simulink model "UAV"  (R2025b)
settings: Solver=ode3  StartTime=0.0  StopTime=inf  FixedStep=Sim.Ts_fisica  RelTol=1e-3
PostLoadFcn:
  | Init
InitFcn:
  | Init
model workspace (MAT data in the model file):
  Mass = 1
undefined symbols (not defined in the file): DiscIntNeverNeededParam, Drone, DWORK0, DWORK1, DWORK10, DWORK11, DWORK12, DWORK13, DWORK14, DWORK15, DWORK16, DWORK17, DWORK18, DWORK19, DWORK2, DWORK20, DWORK21, DWORK22, DWORK23, DWORK24, DWORK3, DWORK4, DWORK5, DWORK6, DWORK7, DWORK8, DWORK9, F, Light, MIL, Sim
libraries: simulink x35, slpidlib x11, vrlib x4, aerolibwind2 x2, sim3dlib x2, uavsim3dlib x2
(part 7 of 8)

== system UAV/Flight Controller Software/Flight Controller Software MIL/Mix Quad-X ==
  Fz : Inport
  T_Phi : Inport  Port=2
  T_Psi : Inport  Port=3
  T_Theta : Inport  Port=4
  M1 : Sum  Inputs=+---
  M2 : Sum  Inputs=+-++
  M3 : Sum  Inputs=++-+
  M4 : Sum  Inputs=+++-
  Saturation{,1..3} (4 alike) : Saturate  UpperLimit=1  LowerLimit=0
  Sqrt{,1..3} (4 alike) : Sqrt
  Motor 1 : Outport
  Motor 2 : Outport  Port=2
  Motor 3 : Outport  Port=3
  Motor 4 : Outport  Port=4
  wires:
  Fz/1 -> M4/1, M3/1, M2/1, M1/1
  T_Phi/1 -> M4/2, M3/2, M2/2, M1/2
  T_Theta/1 -> M4/3, M3/3, M2/3, M1/3
  T_Psi/1 -> M4/4, M3/4, M2/4, M1/4
  M1/1 -> Saturation/1
  M2/1 -> Saturation1/1
  M3/1 -> Saturation2/1
  M4/1 -> Saturation3/1
  Saturation/1 -> Sqrt/1
  Saturation1/1 -> Sqrt1/1
  Saturation2/1 -> Sqrt2/1
  Saturation3/1 -> Sqrt3/1
  Sqrt/1 -> Motor 1/1
  Sqrt1/1 -> Motor 2/1
  Sqrt2/1 -> Motor 3/1
  Sqrt3/1 -> Motor 4/1

== system UAV/Flight Controller Software/Flight Controller Software MIL/State Estimator ==
  " System_Ready" : Inport
  " " : Inport  Port=2
  Bus Selector : BusSelector  OutputSignals=Wb_m,Acc_m,Mag_m,Xe_m,Ve_m,z_m
  MATLAB Function : MATLAB Function  TreatAsAtomicUnit=on  SystemSampleTime=Sim.Ts_pos
  MATLAB Function2 : MATLAB Function  TreatAsAtomicUnit=on  SystemSampleTime=Sim.Ts_control
  Rate Transition{1..4} (4 alike) : RateTransition  OutPortSampleTime=Sim.Ts_pos
  Selector : Selector  InputPortWidth=6  IndexOptions=Index vector (dialog)  Indices=[3]  OutputSizes=1
  Subsystem : Subsystem
  Transpose : Math  Operator=transpose
  Rates : Outport
  Angles : Outport  Port=2
  Pos : Outport  Port=3
  Vel : Outport  Port=4
  DCMbe : Outport  Port=5
  wires:
  Bus Selector/4 -> MATLAB Function/3(gps_pos)  "<Xe_m>"
  " "/1 -> Bus Selector/1
  Bus Selector/1 -> Rates/1, MATLAB Function2/2(gyro_rates)  "<Wb_m>"
  Bus Selector/5 -> MATLAB Function/4(gps_vel)  "<Ve_m>"
  Selector/1 -> MATLAB Function2/4(system_ready), Rate Transition2/1
  Bus Selector/2 -> MATLAB Function2/1(raw_accel_vec), Rate Transition3/1  "<Acc_m>"
  MATLAB Function/1(pos_ned) -> Pos/1
  Subsystem/1(Out1) -> Vel/1
  Bus Selector/3 -> MATLAB Function2/3(mag_body)  "<Mag_m>"
  Bus Selector/6 -> MATLAB Function/5(baro_alt)  "<z_m>"
  Rate Transition3/1 -> MATLAB Function/1(acc_body)
  Rate Transition1/1 -> MATLAB Function/2(DCM_be)
  Rate Transition2/1 -> MATLAB Function/6(system_ready)
  MATLAB Function/2(vel_ned) -> Subsystem/1(vel_ned)
  MATLAB Function2/2(angle_est) -> Angles/1
  Rate Transition4/1 -> DCMbe/1, Subsystem/2(DCMbe)
  " System_Ready"/1 -> Selector/1
  Transpose/1 -> Rate Transition4/1
  MATLAB Function2/3(DCM_be) -> Rate Transition1/1, Transpose/1

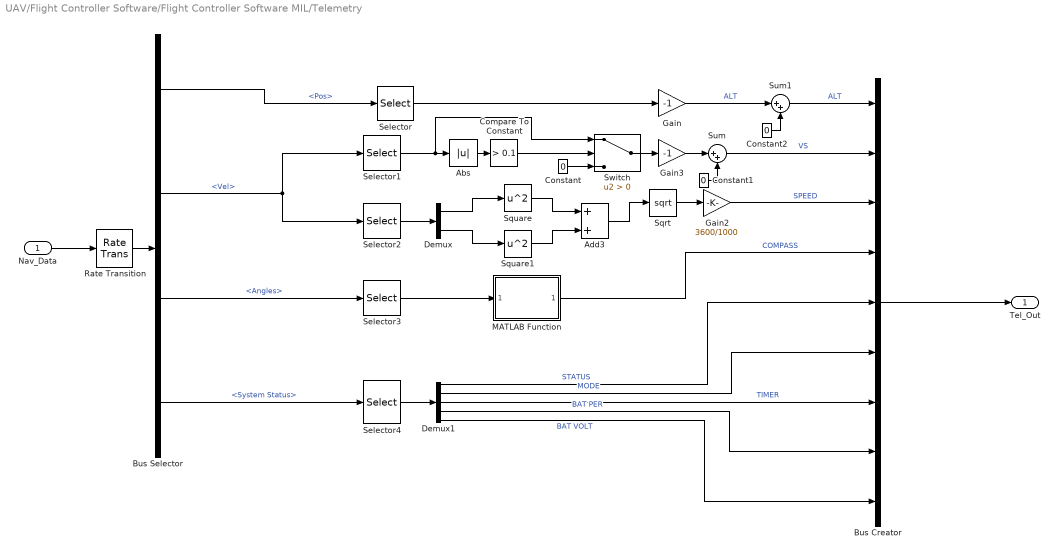
== system UAV/Flight Controller Software/Flight Controller Software MIL/Telemetry ==
  Nav_Data : Inport
  Abs : Abs  SaturateOnIntegerOverflow=off
  Add3 : Sum
  Bus Creator : BusCreator  Inputs=9
  Bus Selector : BusSelector  OutputSignals=Pos,Vel,Angles,System Status
  Compare To Constant : simulink/Logic and Bit Operations/Compare To Constant  relop=>  const=0.1  OutDataTypeStr=boolean
  Constant : Constant  Value=0
  Constant1 : Constant  Value=0
  Constant2 : Constant  Value=0
  Demux : Demux  Outputs=2
  Demux1 : Demux  Outputs=5
  Gain : Gain  Gain=-1
  Gain2 : Gain  Gain=3600/1000
  Gain3 : Gain  Gain=-1
  MATLAB Function : MATLAB Function  TreatAsAtomicUnit=on
  Rate Transition : RateTransition  OutPortSampleTime=Sim.Ts_video
  Selector : Selector  InputPortWidth=3  IndexOptions=Index vector (dialog)  Indices=[3]  OutputSizes=1
  Selector1 : Selector  InputPortWidth=3  IndexOptions=Index vector (dialog)  Indices=[3]  OutputSizes=1
  Selector2 : Selector  InputPortWidth=3  IndexOptions=Index vector (dialog)  Indices=[1 2]  OutputSizes=1
  Selector3 : Selector  InputPortWidth=3  IndexOptions=Index vector (dialog)  Indices=[3]  OutputSizes=1
  Selector4 : Selector  InputPortWidth=6  IndexOptions=Index vector (dialog)  Indices=[1 2 4 5 6]  OutputSizes=1
  Sqrt : Sqrt
  Square : Math  Operator=square  SignedPower=on  RndMeth=Zero
  Square1 : Math  Operator=square  SignedPower=on  RndMeth=Zero
  Sum : Sum  Inputs=|++
  Sum1 : Sum  Inputs=|++
  Switch : Switch  Criteria=u2 > Threshold  SaturateOnIntegerOverflow=off  InputSameDT=off
  "Tel_Out " : Outport
  wires:
  Sum/1 -> Bus Creator/2  "VS"
  Selector/1 -> Gain/1
  Bus Selector/3 -> Selector3/1  "<Angles>"
  MATLAB Function/1(heading) -> Bus Creator/4  "COMPASS"
  Square1/1 -> Add3/2
  Square/1 -> Add3/1
  Add3/1 -> Sqrt/1
  Demux/1 -> Square/1
  Demux/2 -> Square1/1
  Sqrt/1 -> Gain2/1
  Gain2/1 -> Bus Creator/3  "SPEED"
  Rate Transition/1 -> Bus Selector/1
  Nav_Data/1 -> Rate Transition/1
  Bus Selector/1 -> Selector/1  "<Pos>"
  Bus Selector/2 -> Selector2/1, Selector1/1  "<Vel>"
  Selector2/1 -> Demux/1
  Demux1/2 -> Bus Creator/6  "MODE"
  Demux1/1 -> Bus Creator/5  "STATUS"
  Selector3/1 -> MATLAB Function/1(yaw_rad)
  Bus Selector/4 -> Selector4/1  "<System Status>"
  Selector4/1 -> Demux1/1
  Demux1/3 -> Bus Creator/7  "TIMER"
  Demux1/4 -> Bus Creator/8  "BAT PER"
  Demux1/5 -> Bus Creator/9  "BAT VOLT"
  Selector1/1 -> Switch/1, Abs/1
  Abs/1 -> Compare To Constant/1
  Compare To Constant/1 -> Switch/2
  Constant/1 -> Switch/3
  Switch/1 -> Gain3/1
  Gain3/1 -> Sum/1
  Constant1/1 -> Sum/2
  Bus Creator/1 -> "Tel_Out "/1
  Constant2/1 -> Sum1/2
  Gain/1 -> Sum1/1  "ALT"
  Sum1/1 -> Bus Creator/1  "ALT"

== system UAV/Flight Controller Software/Flight Controller Software SIL/__InputSSForSFun__ ==
  Pilot Inputs : Inport
  Power_Status : Inport  Port=2
  Measurements_In : Inport  Port=3
  temporaryBusSelectName_1 : BusSelector  OutputSignals=Roll,Pitch,Yaw,Throttle,Arm/Disarm,Mode
  temporaryBusSelectName_2 : BusSelector  OutputSignals=Volt,Curr
  temporaryBusSelectName_3 : BusSelector  OutputSignals=Ve_m,Xe_m,z_m,Mag_m,Wb_m,Acc_m
  __UniqueOutportName__1__ : Outport
  __UniqueOutportName__2__ : Outport  Port=2
  __UniqueOutportName__3__ : Outport  Port=3
  __UniqueOutportName__4__ : Outport  Port=4
  __UniqueOutportName__5__ : Outport  Port=5
  __UniqueOutportName__6__ : Outport  Port=6
  __UniqueOutportName__7__ : Outport  Port=7
  __UniqueOutportName__8__ : Outport  Port=8
  __UniqueOutportName__9__ : Outport  Port=9
  __UniqueOutportName__10__ : Outport  Port=10
  __UniqueOutportName__11__ : Outport  Port=11
  __UniqueOutportName__12__ : Outport  Port=12
  __UniqueOutportName__13__ : Outport  Port=13
  __UniqueOutportName__14__ : Outport  Port=14
  wires:
  Pilot Inputs/1 -> temporaryBusSelectName_1/1
  Power_Status/1 -> temporaryBusSelectName_2/1
  Measurements_In/1 -> temporaryBusSelectName_3/1
  temporaryBusSelectName_1/1 -> __UniqueOutportName__1__/1  "<Roll>"
  temporaryBusSelectName_1/2 -> __UniqueOutportName__2__/1  "<Pitch>"
  temporaryBusSelectName_1/3 -> __UniqueOutportName__3__/1  "<Yaw>"
  temporaryBusSelectName_1/4 -> __UniqueOutportName__4__/1  "<Throttle>"
  temporaryBusSelectName_1/5 -> __UniqueOutportName__5__/1  "<Arm/Disarm>"
  temporaryBusSelectName_1/6 -> __UniqueOutportName__6__/1  "<Mode>"
  temporaryBusSelectName_2/1 -> __UniqueOutportName__7__/1  "<Volt>"
  temporaryBusSelectName_2/2 -> __UniqueOutportName__8__/1  "<Curr>"
  temporaryBusSelectName_3/1 -> __UniqueOutportName__9__/1  "<Ve_m>"
  temporaryBusSelectName_3/2 -> __UniqueOutportName__10__/1  "<Xe_m>"
  temporaryBusSelectName_3/3 -> __UniqueOutportName__11__/1  "<z_m>"
  temporaryBusSelectName_3/4 -> __UniqueOutportName__12__/1  "<Mag_m>"
  temporaryBusSelectName_3/5 -> __UniqueOutportName__13__/1  "<Wb_m>"
  temporaryBusSelectName_3/6 -> __UniqueOutportName__14__/1  "<Acc_m>"

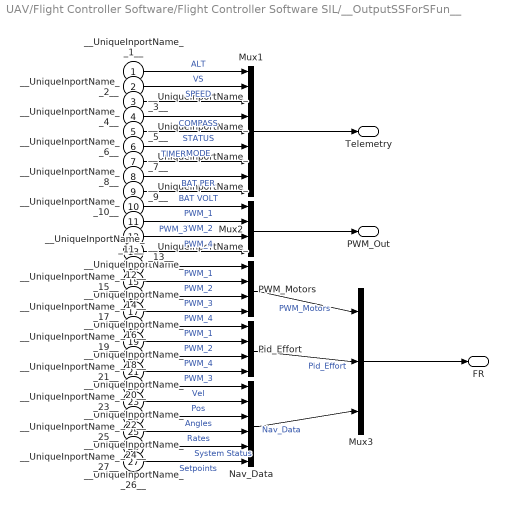
== system UAV/Flight Controller Software/Flight Controller Software SIL/__OutputSSForSFun__ ==
  __UniqueInportName__1__ : Inport
  __UniqueInportName__2__ : Inport  Port=2
  __UniqueInportName__3__ : Inport  Port=3
  __UniqueInportName__4__ : Inport  Port=4
  __UniqueInportName__5__ : Inport  Port=5
  __UniqueInportName__6__ : Inport  Port=6
  __UniqueInportName__7__ : Inport  Port=7
  __UniqueInportName__8__ : Inport  Port=8
  __UniqueInportName__9__ : Inport  Port=9
  __UniqueInportName__10__ : Inport  Port=10
  __UniqueInportName__11__ : Inport  Port=11
  __UniqueInportName__12__ : Inport  Port=12
  __UniqueInportName__13__ : Inport  Port=13
  __UniqueInportName__14__ : Inport  Port=14
  __UniqueInportName__15__ : Inport  Port=15
  __UniqueInportName__16__ : Inport  Port=16
  __UniqueInportName__17__ : Inport  Port=17
  __UniqueInportName__18__ : Inport  Port=18
  __UniqueInportName__19__ : Inport  Port=19
  __UniqueInportName__20__ : Inport  Port=20
  __UniqueInportName__21__ : Inport  Port=21
  __UniqueInportName__22__ : Inport  Port=22
  __UniqueInportName__23__ : Inport  Port=23
  __UniqueInportName__24__ : Inport  Port=24
  __UniqueInportName__25__ : Inport  Port=25
  __UniqueInportName__26__ : Inport  Port=26
  __UniqueInportName__27__ : Inport  Port=27
  Mux1 : BusCreator  Inputs=9
  Mux2 : BusCreator  Inputs=4
  Mux3 : BusCreator  Inputs=3
  Nav_Data : BusCreator  Inputs=6
  PWM_Motors : BusCreator  Inputs=4
  Pid_Effort : BusCreator  Inputs=4
  "Telemetry " : Outport
  PWM_Out : Outport  Port=2
  FR : Outport  Port=3
  wires:
  __UniqueInportName__1__/1 -> Mux1/1  "ALT"
  __UniqueInportName__2__/1 -> Mux1/2  "VS"
  __UniqueInportName__3__/1 -> Mux1/3  "SPEED"
  __UniqueInportName__4__/1 -> Mux1/4  "COMPASS"
  __UniqueInportName__5__/1 -> Mux1/5  "STATUS"
  __UniqueInportName__6__/1 -> Mux1/6  "MODE"
  __UniqueInportName__7__/1 -> Mux1/7  "TIMER"
  __UniqueInportName__8__/1 -> Mux1/8  "BAT PER"
  __UniqueInportName__9__/1 -> Mux1/9  "BAT VOLT"
  Mux1/1 -> "Telemetry "/1
  __UniqueInportName__10__/1 -> Mux2/1  "PWM_1"
  __UniqueInportName__11__/1 -> Mux2/2  "PWM_2"
  __UniqueInportName__12__/1 -> Mux2/3  "PWM_3"
  __UniqueInportName__13__/1 -> Mux2/4  "PWM_4"
  Mux2/1 -> PWM_Out/1
  __UniqueInportName__14__/1 -> PWM_Motors/1  "PWM_1"
  __UniqueInportName__15__/1 -> PWM_Motors/2  "PWM_2"
  __UniqueInportName__16__/1 -> PWM_Motors/3  "PWM_3"
  __UniqueInportName__17__/1 -> PWM_Motors/4  "PWM_4"
  __UniqueInportName__18__/1 -> Pid_Effort/1  "PWM_1"
  __UniqueInportName__19__/1 -> Pid_Effort/2  "PWM_2"
  __UniqueInportName__20__/1 -> Pid_Effort/3  "PWM_4"
  __UniqueInportName__21__/1 -> Pid_Effort/4  "PWM_3"
  __UniqueInportName__22__/1 -> Nav_Data/1  "Vel"
  __UniqueInportName__23__/1 -> Nav_Data/2  "Pos"
  __UniqueInportName__24__/1 -> Nav_Data/3  "Angles"
  __UniqueInportName__25__/1 -> Nav_Data/4  "Rates"
  __UniqueInportName__26__/1 -> Nav_Data/5  "System Status"
  __UniqueInportName__27__/1 -> Nav_Data/6  "Setpoints"
  PWM_Motors/1 -> Mux3/1  "PWM_Motors"
  Pid_Effort/1 -> Mux3/2  "Pid_Effort"
  Nav_Data/1 -> Mux3/3  "Nav_Data"
  Mux3/1 -> FR/1

== system UAV/Pilot Interface/Real_Receiver_Driver /Command Acquisition ==
  Add : Sum  Inputs=+++
  Bias : Bias  Bias=1  SaturateOnIntegerOverflow=off
  Bus Creator : BusCreator  Inputs=6
  Constant : Constant  Value=3
  Gain : Gain
  Gain1 : Gain  Gain=2
  Gain2 : Gain  Gain=3
  Gain4 : Gain  Gain=0.5
  HotasX56 FlightStick : vrlib/Joystick Input  joyid=1  adjustports=on  forcefeed=off
  HotasX56 Throttle : vrlib/Joystick Input  joyid=2  adjustports=on  forcefeed=off
  Subsystem : Subsystem
  Subsystem1 : Subsystem
  Subsystem2 : Subsystem
  Subsystem3 : Subsystem
  Subsystem4 : Subsystem
  Switch : Switch  Criteria=u2 > Threshold  SaturateOnIntegerOverflow=off  InputSameDT=off
  Pilot Inputs : Outport
  wires:
  Bus Creator/1 -> Pilot Inputs/1
  Gain/1 -> Add/1
  Subsystem4/34(M1) -> Gain/1
  Constant/1 -> Switch/3
  HotasX56 FlightStick/3 -> Subsystem2/1(In1)
  Gain4/1 -> Bus Creator/4  "Throttle"
  Subsystem4/33(SLD) -> Bus Creator/5  "Arm/Disarm"
  Switch/1 -> Bus Creator/6  "Mode"
  Gain1/1 -> Add/2
  Gain2/1 -> Add/3
  Add/1 -> Switch/1, Switch/2
  Bias/1 -> Gain4/1
  Subsystem/3(Yaw) -> Bus Creator/3  "Yaw"
  Subsystem/2(Pitch) -> Bus Creator/2  "Pitch"
  HotasX56 FlightStick/1 -> Subsystem/1(In1)
  Subsystem3/3(F) -> Bias/1
  Subsystem/1(Roll) -> Bus Creator/1  "Roll"
  HotasX56 Throttle/1 -> Subsystem3/1(In1)
  HotasX56 FlightStick/2 -> Subsystem1/1(In1)
  HotasX56 Throttle/2 -> Subsystem4/1(In1)
  Subsystem4/36(S1) -> Gain2/1
  Subsystem4/35(M2) -> Gain1/1

== system UAV/Pilot Interface/Real_Receiver_Driver /Flight Data Display ==
  Telemetry : Inport
  Bus Selector : BusSelector  OutputSignals=ALT,VS,SPEED,COMPASS,STATUS,MODE,TIMER,BAT PER,BAT VOLT
  Subsystem : Subsystem
  Terminator{2..10} (9 alike) : Terminator
  wires:
  Telemetry/1 -> Bus Selector/1
  Bus Selector/1 -> Terminator2/1  "<ALT>"
  Bus Selector/2 -> Terminator3/1  "<VS>"
  Bus Selector/3 -> Terminator4/1  "<SPEED>"
  Bus Selector/4 -> Terminator5/1  "<COMPASS>"
  Bus Selector/5 -> Terminator6/1  "<STATUS>"
  Bus Selector/6 -> Terminator7/1  "<MODE>"
  Bus Selector/8 -> Terminator9/1  "<BAT PER>"
  Bus Selector/9 -> Terminator10/1  "<BAT VOLT>"
  Bus Selector/7 -> Subsystem/1(seg)  "<TIMER>"
  Subsystem/1(MM:SS) -> Terminator8/1

== system UAV/Pilot Interface/SIM_Flightstick_HotasX56 /Command Acquisition ==
  Add : Sum  Inputs=+++
  Bias : Bias  Bias=1  SaturateOnIntegerOverflow=off
  Bus Creator : BusCreator  Inputs=6
  Constant : Constant  Value=3
  Gain : Gain
  Gain1 : Gain  Gain=2
  Gain2 : Gain  Gain=3
  Gain4 : Gain  Gain=0.5
  HotasX56 FlightStick : vrlib/Joystick Input  joyid=1  adjustports=on  forcefeed=off
  HotasX56 Throttle : vrlib/Joystick Input  joyid=2  adjustports=on  forcefeed=off
  Subsystem : Subsystem
  Subsystem1 : Subsystem
  Subsystem2 : Subsystem
  Subsystem3 : Subsystem
  Subsystem4 : Subsystem
  Switch : Switch  Criteria=u2 > Threshold  SaturateOnIntegerOverflow=off  InputSameDT=off
  Pilot Inputs : Outport
  wires:
  Bus Creator/1 -> Pilot Inputs/1
  Gain/1 -> Add/1
  Subsystem4/34(M1) -> Gain/1
  Constant/1 -> Switch/3
  HotasX56 FlightStick/3 -> Subsystem2/1(In1)
  Gain4/1 -> Bus Creator/4  "Throttle"
  Subsystem4/33(SLD) -> Bus Creator/5  "Arm/Disarm"
  Switch/1 -> Bus Creator/6  "Mode"
  Gain1/1 -> Add/2
  Gain2/1 -> Add/3
  Add/1 -> Switch/1, Switch/2
  Bias/1 -> Gain4/1
  Subsystem/3(Yaw) -> Bus Creator/3  "Yaw"
  Subsystem/2(Pitch) -> Bus Creator/2  "Pitch"
  HotasX56 FlightStick/1 -> Subsystem/1(In1)
  Subsystem3/3(F) -> Bias/1
  Subsystem/1(Roll) -> Bus Creator/1  "Roll"
  HotasX56 Throttle/1 -> Subsystem3/1(In1)
  HotasX56 FlightStick/2 -> Subsystem1/1(In1)
  HotasX56 Throttle/2 -> Subsystem4/1(In1)
  Subsystem4/36(S1) -> Gain2/1
  Subsystem4/35(M2) -> Gain1/1

== system UAV/Pilot Interface/SIM_Flightstick_HotasX56 /Flight Data Display ==
  Telemetry : Inport
  Bus Selector : BusSelector  OutputSignals=ALT,VS,SPEED,COMPASS,STATUS,MODE,TIMER,BAT PER,BAT VOLT
  Subsystem : Subsystem
  Terminator{2..10} (9 alike) : Terminator
  wires:
  Telemetry/1 -> Bus Selector/1
  Bus Selector/1 -> Terminator2/1  "<ALT>"
  Bus Selector/2 -> Terminator3/1  "<VS>"
  Bus Selector/3 -> Terminator4/1  "<SPEED>"
  Bus Selector/4 -> Terminator5/1  "<COMPASS>"
  Bus Selector/5 -> Terminator6/1  "<STATUS>"
  Bus Selector/6 -> Terminator7/1  "<MODE>"
  Bus Selector/8 -> Terminator9/1  "<BAT PER>"
  Bus Selector/9 -> Terminator10/1  "<BAT VOLT>"
  Bus Selector/7 -> Subsystem/1(seg)  "<TIMER>"
  Subsystem/1(MM:SS) -> Terminator8/1

== system UAV/Vehicle Interface/Real_Hardware_Drivers/ADC ==
  In1 : Inport
  Battery_Curr : Inport  Port=2
  Abs : Abs  SaturateOnIntegerOverflow=off
  Abs1 : Abs  SaturateOnIntegerOverflow=off
  Band-Limited White Noise : simulink/Sources/Band-Limited White Noise  Cov=Drone.Sensors.Voltage.NoisePower  Ts=Sim.Ts_logic  seed=[23341]
  Band-Limited White Noise1 : simulink/Sources/Band-Limited White Noise  Cov=Drone.Sensors.Current.NoisePower  Ts=Sim.Ts_logic  seed=[23341]
  Quantizer : Quantizer  QuantizationInterval=Drone.Sensors.Voltage.Quantum
  Quantizer1 : Quantizer  QuantizationInterval=Drone.Sensors.Current.Quantum
  Sum : Sum  Inputs=|++
  Sum1 : Sum  Inputs=|++
  Unit Delay1 : UnitDelay  InitialCondition=16.8  SampleTime=-1  HasFrameUpgradeWarning=on
  Unit Delay2 : UnitDelay  InitialCondition=16.8  SampleTime=-1  HasFrameUpgradeWarning=on
  Zero-Order Hold : ZeroOrderHold  SampleTime=Sim.Ts_logic
  Zero-Order Hold1 : ZeroOrderHold  SampleTime=Sim.Ts_logic
  Out1 : Outport
  Out2 : Outport  Port=2
  wires:
  In1/1 -> Zero-Order Hold/1
  Zero-Order Hold/1 -> Sum/1
  Sum/1 -> Abs/1
  Band-Limited White Noise/1 -> Sum/2
  Battery_Curr/1 -> Zero-Order Hold1/1
  Sum1/1 -> Abs1/1
  Quantizer/1 -> Unit Delay1/1
  Zero-Order Hold1/1 -> Sum1/1
  Band-Limited White Noise1/1 -> Sum1/2
  Quantizer1/1 -> Unit Delay2/1
  Unit Delay1/1 -> Out1/1
  Unit Delay2/1 -> Out2/1
  Abs/1 -> Quantizer/1
  Abs1/1 -> Quantizer1/1

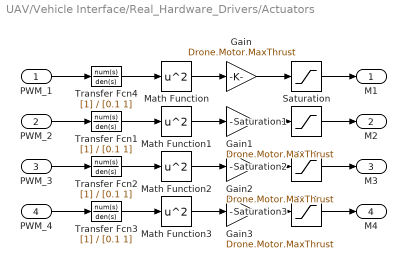
== system UAV/Vehicle Interface/Real_Hardware_Drivers/Actuators ==
  PWM_1 : Inport
  PWM_2 : Inport  Port=2
  PWM_3 : Inport  Port=3
  PWM_4 : Inport  Port=4
  Gain{,1..3} (4 alike) : Gain  Gain=Drone.Motor.MaxThrust
  Math Function{,1..3} (4 alike) : Math  Operator=square
  Saturation{,1..3} (4 alike) : Saturate  UpperLimit=Drone.Motor.MaxThrust  LowerLimit=Drone.Motor.MinThrust
  Transfer Fcn{1..4} (4 alike) : TransferFcn  Denominator=[0.1 1]
  M1 : Outport
  M2 : Outport  Port=2
  M3 : Outport  Port=3
  M4 : Outport  Port=4
  wires:
  PWM_1/1 -> Transfer Fcn4/1
  PWM_2/1 -> Transfer Fcn1/1
  PWM_3/1 -> Transfer Fcn2/1
  PWM_4/1 -> Transfer Fcn3/1
  Transfer Fcn4/1 -> Math Function/1
  Transfer Fcn1/1 -> Math Function1/1
  Transfer Fcn2/1 -> Math Function2/1
  Transfer Fcn3/1 -> Math Function3/1
  Gain/1 -> Saturation/1
  Saturation/1 -> M1/1
  Saturation1/1 -> M2/1
  Saturation2/1 -> M3/1
  Saturation3/1 -> M4/1
  Gain1/1 -> Saturation1/1
  Gain2/1 -> Saturation2/1
  Gain3/1 -> Saturation3/1
  Math Function/1 -> Gain/1
  Math Function1/1 -> Gain1/1
  Math Function2/1 -> Gain2/1
  Math Function3/1 -> Gain3/1

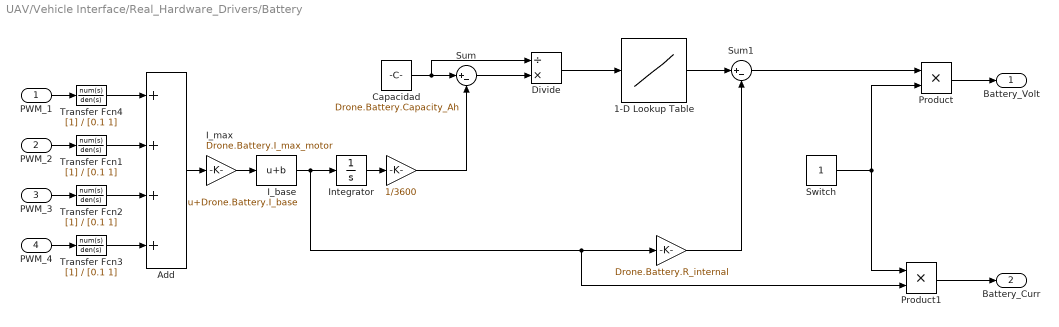
== system UAV/Vehicle Interface/Real_Hardware_Drivers/Battery ==
  PWM_1 : Inport
  PWM_2 : Inport  Port=2
  PWM_3 : Inport  Port=3
  PWM_4 : Inport  Port=4
  " " : Gain  Gain=1/3600
  "  " : Gain  Gain=Drone.Battery.R_internal
  1-D Lookup Table : Lookup_n-D  NumberOfTableDimensions=1  BreakpointsForDimension1=Drone.Battery.DischargeCurve_Cap  Table=Drone.Battery.DischargeCurve_Vol  InternalRulePriority=Speed  RndMeth=Simplest
  Add : Sum  Inputs=++++
  Capacidad : Constant  Value=Drone.Battery.Capacity_Ah
  Divide : Product  Inputs=/*
  I_base : Bias  Bias=Drone.Battery.I_base  SaturateOnIntegerOverflow=off
  I_max : Gain  Gain=Drone.Battery.I_max_motor
  Integrator : Integrator
  Product : Product
  Product1 : Product
  Sum : Sum  Inputs=|+-
  Sum1 : Sum  Inputs=|+-
  Switch : Constant
  Transfer Fcn{1..4} (4 alike) : TransferFcn  Denominator=[0.1 1]
  Battery_Volt : Outport
  Battery_Curr : Outport  Port=2
  wires:
  Transfer Fcn1/1 -> Add/2
  Transfer Fcn3/1 -> Add/4
  Add/1 -> I_max/1
  Transfer Fcn4/1 -> Add/1
  Transfer Fcn2/1 -> Add/3
  PWM_1/1 -> Transfer Fcn4/1
  PWM_2/1 -> Transfer Fcn1/1
  PWM_3/1 -> Transfer Fcn2/1
  PWM_4/1 -> Transfer Fcn3/1
  I_max/1 -> I_base/1
  Integrator/1 -> " "/1
  Capacidad/1 -> Divide/1, Sum/1
  " "/1 -> Sum/2
  Sum/1 -> Divide/2
  Divide/1 -> 1-D Lookup Table/1
  1-D Lookup Table/1 -> Sum1/1
  "  "/1 -> Sum1/2
  I_base/1 -> Product1/2, "  "/1, Integrator/1
  Switch/1 -> Product1/1, Product/2
  Product1/1 -> Battery_Curr/1
  Product/1 -> Battery_Volt/1
  Sum1/1 -> Product/1

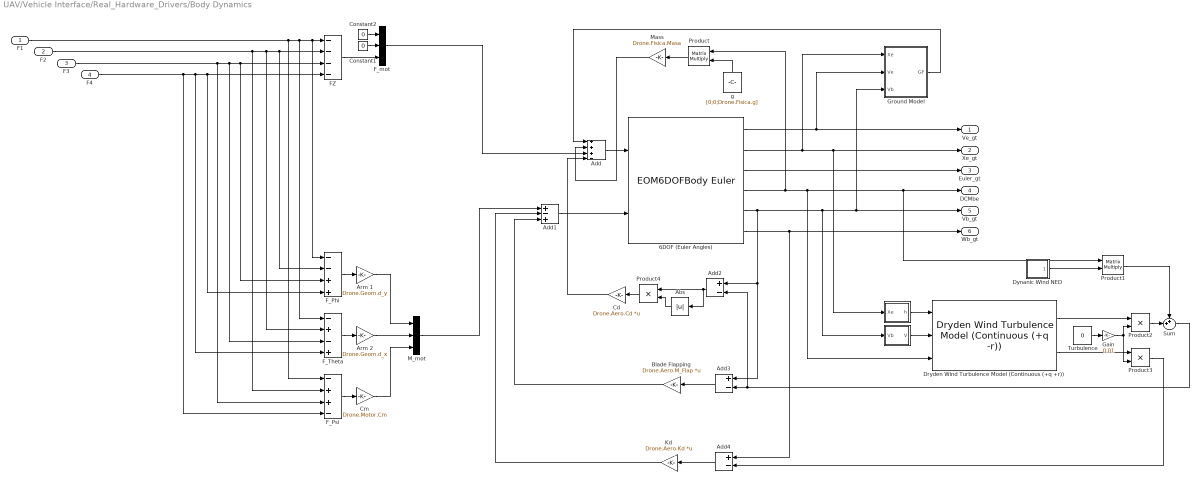
== system UAV/Vehicle Interface/Real_Hardware_Drivers/Body Dynamics ==
  F1 : Inport
  F2 : Inport  Port=2
  F3 : Inport  Port=3
  F4 : Inport  Port=4
  " " : Subsystem
  "  " : Subsystem
  6DOF (Euler Angles) : EOM6DOFBodyEuler  xme_0=Env.Pos.Init_NED  mass_0=Drone.Fisica.Masa  inertia=Drone.Fisica.InertiaMatrix
  Abs : Abs  SaturateOnIntegerOverflow=off
  Add : Sum  Inputs=+++-
  Add1 : Sum  Inputs=+-+
  Add2 : Sum  Inputs=+-
  Add3 : Sum  Inputs=+-
  Add4 : Sum  Inputs=+-
  Arm 1 : Gain  Gain=Drone.Geom.d_y
  Arm 2 : Gain  Gain=Drone.Geom.d_x
  Blade Flapping : Gain  Gain=Drone.Aero.M_Flap  Multiplication=Matrix(K*u) (u vector)
  Cd : Gain  Gain=Drone.Aero.Cd  Multiplication=Matrix(K*u) (u vector)
  Cm : Gain  Gain=Drone.Motor.Cm
  Constant1 : Constant  Value=0
  Constant2 : Constant  Value=0
  Dryden Wind Turbulence Model (Continuous (+q +r)) : aerolibwind2/Dryden Wind Turbulence Model  (Continuous (+q -r))  units=Metric (MKS)  spec=MIL-F-8785C  model=Continuous Dryden (+q +r)  W20=Env.Viento.Intensidad_Max  Wdeg=0  TurbProb=10^-2 - Light  L_high=533.4  Wingspan=0.318  ts=1/100  Seed=[23341 23342 23343 23344]  T_on=on
      settings: LibrarySourceBlock=|
      | aerolibwind2/Dryden Wind Turbulence Model
      | (Continuous (+q +r))
  Dynanic Wind NED : Subsystem
  FZ : Sum  Inputs=----
  F_Phi : Sum  Inputs=--++
  F_Psi : Sum  Inputs=-++-
  F_Theta : Sum  Inputs=-+-+
  F_mot : Mux  Inputs=3
  Gain : Gain  Gain=0.01
  Ground Model : Subsystem
  Kd : Gain  Gain=Drone.Aero.Kd  Multiplication=Matrix(K*u) (u vector)
  M_mot : Mux  Inputs=3
  Mass : Gain  Gain=Drone.Fisica.Masa
  Product : Product  Multiplication=Matrix(*)
  Product1 : Product  Multiplication=Matrix(*)
  Product2 : Product
  Product3 : Product
  Product4 : Product
  Sum : Sum  Inputs=++|
  Turbulence : Constant  Value=0
  g : Constant  Value=[0;0;Drone.Fisica.g]
  Ve_gt : Outport
  Xe_gt : Outport  Port=2
  Euler_gt : Outport  Port=3
  DCMbe : Outport  Port=4
  Vb_gt : Outport  Port=5
  Wb_gt : Outport  Port=6
  wires:
  F_Phi/1 -> Arm 1/1
  F_Psi/1 -> Cm/1
  F_Theta/1 -> Arm 2/1
  F4/1 -> F_Psi/4, F_Theta/4, F_Phi/4, FZ/4
  F3/1 -> F_Psi/3, F_Theta/3, F_Phi/3, FZ/3
  F2/1 -> F_Psi/2, F_Theta/2, F_Phi/2, FZ/2
  F1/1 -> F_Psi/1, F_Theta/1, F_Phi/1, FZ/1
  Constant1/1 -> F_mot/2
  Constant2/1 -> F_mot/1
  Arm 1/1 -> M_mot/1
  Arm 2/1 -> M_mot/2
  Cm/1 -> M_mot/3
  6DOF (Euler Angles)/6 -> Add4/1, Wb_gt/1
  6DOF (Euler Angles)/5 -> Add2/1, Add3/1, " "/1(Vb), Ground Model/3(Vb), Vb_gt/1
  Add/1 -> 6DOF (Euler Angles)/1
  Add1/1 -> 6DOF (Euler Angles)/2
  M_mot/1 -> Add1/1
  Blade Flapping/1 -> Add1/3
  Kd/1 -> Add1/2
  F_mot/1 -> Add/3
  Cd/1 -> Add/4
  Product/1 -> Mass/1
  Mass/1 -> Add/2
  g/1 -> Product/2
  6DOF (Euler Angles)/4 -> Dryden Wind Turbulence Model (Continuous (+q +r))/3, Product1/1, DCMbe/1, Product/1
  6DOF (Euler Angles)/1 -> Ve_gt/1, Ground Model/2(Ve)
  6DOF (Euler Angles)/3 -> Euler_gt/1
  Ground Model/1(GF) -> Add/1
  6DOF (Euler Angles)/2 -> "  "/1(Xe), Xe_gt/1, Ground Model/1(Xe)
  FZ/1 -> F_mot/3
  " "/1(V) -> Dryden Wind Turbulence Model (Continuous (+q +r))/2
  "  "/1(h) -> Dryden Wind Turbulence Model (Continuous (+q +r))/1
  Dryden Wind Turbulence Model (Continuous (+q +r))/1 -> Product2/1
  Add3/1 -> Blade Flapping/1
  Add4/1 -> Kd/1
  Dryden Wind Turbulence Model (Continuous (+q +r))/2 -> Product3/1
  Product1/1 -> Sum/1
  Product2/1 -> Sum/2
  Sum/1 -> Add2/2, Add3/2
  Dynanic Wind NED/1(Out1) -> Product1/2
  Turbulence/1 -> Gain/1
  Gain/1 -> Product2/2, Product3/2
  Product3/1 -> Add4/2
  Product4/1 -> Cd/1
  Add2/1 -> Abs/1, Product4/1
  Abs/1 -> Product4/2

== system UAV/Vehicle Interface/Real_Hardware_Drivers/ESC_Quantization_Model ==
  In1 : Inport
  Bias : Bias  Bias=1000  SaturateOnIntegerOverflow=off
  Bias1 : Bias  Bias=-1000  SaturateOnIntegerOverflow=off
  Data Type Conversion : DataTypeConversion  OutDataTypeStr=uint16  SaturateOnIntegerOverflow=off  RndMeth=Floor  LockScale=on
  Data Type Conversion1 : DataTypeConversion  OutDataTypeStr=double  SaturateOnIntegerOverflow=off  RndMeth=Floor  LockScale=on
  Gain : Gain  Gain=1000
  Gain1 : Gain  Gain=1/1000
  Out1 : Outport
  wires:
  Bias/1 -> Data Type Conversion/1
  Data Type Conversion/1 -> Data Type Conversion1/1
  Bias1/1 -> Gain1/1
  Data Type Conversion1/1 -> Bias1/1
  Gain1/1 -> Out1/1
  Gain/1 -> Bias/1
  In1/1 -> Gain/1

== system UAV/Vehicle Interface/Real_Hardware_Drivers/Flight Recorder ==
  Nav_Data : Inport
  PID_Effort : Inport  Port=2
  Motor_PWM : Inport  Port=3
  To Workspace : ToWorkspace  VariableName=Log_Nav  SaveFormat=Structure With Time  SampleTime=-1
  To Workspace1 : ToWorkspace  VariableName=PID_Effort  SaveFormat=Structure With Time  SampleTime=-1
  To Workspace2 : ToWorkspace  VariableName=Motor_PWM  SaveFormat=Structure With Time  SampleTime=-1
  wires:
  PID_Effort/1 -> To Workspace1/1
  Motor_PWM/1 -> To Workspace2/1
  Nav_Data/1 -> To Workspace/1

== system UAV/Vehicle Interface/Real_Hardware_Drivers/Sensors ==
  Ve : Inport
  Xe : Inport  Port=2
  Euler : Inport  Port=3
  DCMbe : Inport  Port=4
  Vb : Inport  Port=5
  Wb : Inport  Port=6
  Barometer : Subsystem
  GPS : Subsystem
  IMU : Subsystem
  Magnetometer : Subsystem
  Ve_m : Outport
  Xe_m : Outport  Port=2
  z_m : Outport  Port=3
  Mag_m : Outport  Port=4
  Gyro_m : Outport  Port=5
  Acc_m : Outport  Port=6
  "Euler_gt " : Outport  Port=7
  "Vb_gt " : Outport  Port=8
  Xe_gt : Outport  Port=9
  Ve_gt : Outport  Port=10
  wires:
  Euler/1 -> "Euler_gt "/1
  DCMbe/1 -> IMU/1(DCMbe), Magnetometer/1(DCMbe)
  Vb/1 -> IMU/2(Vb_gt), "Vb_gt "/1
  Wb/1 -> IMU/3(Wb_gt)
  IMU/2(Gyro_m) -> Gyro_m/1
  IMU/1(Acc_m) -> Acc_m/1
  Xe/1 -> Barometer/1(Xe), Xe_gt/1, GPS/2(Xe)
  Ve/1 -> Ve_gt/1, GPS/1(Ve)
  GPS/1(Ve_m) -> Ve_m/1
  GPS/2(Xe_m) -> Xe_m/1
  Barometer/1(z_m) -> z_m/1
  Magnetometer/1(Mag_m) -> Mag_m/1

== system UAV/Vehicle Interface/Real_Hardware_Drivers/Visualization ==
  Ground Truth : Inport
  Bus Selector : BusSelector  OutputSignals=Xe_gt,Euler_gt
  NED to ENU : Subsystem
  Simulation 3D Scene Configuration : sim3dlib/Simulation 3D Scene Configuration  Priority=0  ProjectFormat=Default Scenes  SceneDesc=US city block  ProjectName=C:\Program Files\MATLAB\R2025b\toolbox\shared\sim3d_projects\automotive_project_windows\UE\WindowsNoEditor\VehicleSimulation.exe  ScenePath=/Game/Maps/USCityBlock  EnableOpenDRIVE=off  vehTagList={'Custom';'Scene Origin';'SimulinkVehicle1'}  vehTag=SimulinkVehicle1  AttachedCameraRelativeTranslation=[0 0 0]  FreeCameraDefaultInitialTranslation=[-6, 0, 2]  AttachedCameraRelativeRotation=[0 0 0]  FreeCameraDefaultInitialRotation=[0, -15, 0]  ViewpointName=Custom  FreeCameraInitialTranslation=[0, 0, 0]  ViewpointTranslation=[0, 0, 0]  FreeCameraInitialRotation=[0, 0, 0]  ViewpointRotation=[0, 0, 0]  OpVisEn=off  Ts=1/50  EnableWindow=on  EnableRemoteAccess=off  EnableWeather=off  SunAzimuth=90  SunAltitude=40.0  EnableGeospatialSun=off  Latitude=0  Longitude=0  Date=2023-01-01  Time=10:30:00  GeoTimeZone=-5.0  SunDaylightSaving=off  wind=1  clouds=10  EnableVolumetricClouds=off  CloudCoverage=0  CloudAltitude=6  fog=0  rain=0  RaindropsEffect=off  SnowDensity=0  EnableGeospatial=off  TilesetSource=Earth terrain  UseTrueOrigin=off  OriginHeight=200  OriginLatitude=40.744652  OriginLongitude=-73.988864  MapStyle=Aerial  AdditionalAssetIDs=[]  UseAdvancedSunSky=off  SolarTime=11  TimeZone=-5  Day=21  Month=9  Year=2022  UseDaylightSavingTime=on  DSTStartDay=10  DSTStartMonth=3  DSTEndDay=3  DSTEndMonth=11  DSTSwitchHour=2  sensorTag=MainCamera2  sensorId=2  sensorName=MainCamera2  mountLoc=Origin  offsetFlag=off  tmountOffset=[0, 0, 0]  rmountOffset=[0, 0, 0]  HorizontalResolution=1280  VerticalResolution=720  HorizontalFOV=60  mountPoint=[0 0 0]  mountOrientation=[0 0 0]  aMode=4  ID=2  GeoTrigger=Inactive  ViewNameList={'Custom'}  ViewTranslationList={'[0 0 0]'}  ViewRotationList={'[0 0 0]'}
      settings: LibrarySourceBlock=uavsim3dlib/Simulation 3D Scene Configuration
  Simulation 3D UAV Vehicle1 : uavsim3dlib/Simulation 3D UAV Vehicle  Priority=-1  Mesh=Quadrotor  MeshPath=/MathWorksUAVContent/UAVs/Quadrotor/Quadrotor.Quadrotor  Color=Black  ActorName=SimulinkVehicle2  UseGlobalFrame=off  InitialTranslation=[0 0 0]  InitialRotation=[0 0 0]  InitialTranslationGlobal=[0 0 0]  InitialGeoOrigin=[0 0 0]  InitialRotationGlobal=[0 0 0]  SampleTime=1/50  ActorType=SimulinkVehicle  ID=2  aMode=4  ActorTag=SimulinkVehicle2
  wires:
  NED to ENU/1(T_ENU) -> Simulation 3D UAV Vehicle1/1
  NED to ENU/2(R_ENU) -> Simulation 3D UAV Vehicle1/2
  Ground Truth/1 -> Bus Selector/1
  Bus Selector/1 -> NED to ENU/1(T_NED)  "<Xe_gt>"
  Bus Selector/2 -> NED to ENU/2(R_NED)  "<Euler_gt>"

== system UAV/Vehicle Interface/Sim_Plant_Model/ADC ==
  In1 : Inport
  Battery_Curr : Inport  Port=2
  Abs : Abs  SaturateOnIntegerOverflow=off
  Abs1 : Abs  SaturateOnIntegerOverflow=off
  Band-Limited White Noise : simulink/Sources/Band-Limited White Noise  Cov=Drone.Sensors.Voltage.NoisePower  Ts=Sim.Ts_logic  seed=[23341]
  Band-Limited White Noise1 : simulink/Sources/Band-Limited White Noise  Cov=Drone.Sensors.Current.NoisePower  Ts=Sim.Ts_logic  seed=[23341]
  Quantizer : Quantizer  QuantizationInterval=Drone.Sensors.Voltage.Quantum
  Quantizer1 : Quantizer  QuantizationInterval=Drone.Sensors.Current.Quantum
  Sum : Sum  Inputs=|++
  Sum1 : Sum  Inputs=|++
  Unit Delay1 : UnitDelay  InitialCondition=16.8  SampleTime=-1  HasFrameUpgradeWarning=on
  Unit Delay2 : UnitDelay  InitialCondition=16.8  SampleTime=-1  HasFrameUpgradeWarning=on
  Zero-Order Hold : ZeroOrderHold  SampleTime=Sim.Ts_logic
  Zero-Order Hold1 : ZeroOrderHold  SampleTime=Sim.Ts_logic
  Out1 : Outport
  Out2 : Outport  Port=2
  wires:
  In1/1 -> Zero-Order Hold/1
  Zero-Order Hold/1 -> Sum/1
  Sum/1 -> Abs/1
  Band-Limited White Noise/1 -> Sum/2
  Battery_Curr/1 -> Zero-Order Hold1/1
  Sum1/1 -> Abs1/1
  Quantizer/1 -> Unit Delay1/1
  Zero-Order Hold1/1 -> Sum1/1
  Band-Limited White Noise1/1 -> Sum1/2
  Quantizer1/1 -> Unit Delay2/1
  Unit Delay1/1 -> Out1/1
  Unit Delay2/1 -> Out2/1
  Abs/1 -> Quantizer/1
  Abs1/1 -> Quantizer1/1

== system UAV/Vehicle Interface/Sim_Plant_Model/Actuators ==
  PWM_1 : Inport
  PWM_2 : Inport  Port=2
  PWM_3 : Inport  Port=3
  PWM_4 : Inport  Port=4
  Gain{,1..3} (4 alike) : Gain  Gain=Drone.Motor.MaxThrust
  Math Function{,1..3} (4 alike) : Math  Operator=square
  Saturation{,1..3} (4 alike) : Saturate  UpperLimit=Drone.Motor.MaxThrust  LowerLimit=Drone.Motor.MinThrust
  Transfer Fcn{1..4} (4 alike) : TransferFcn  Denominator=[0.1 1]
  M1 : Outport
  M2 : Outport  Port=2
  M3 : Outport  Port=3
  M4 : Outport  Port=4
  wires:
  PWM_1/1 -> Transfer Fcn4/1
  PWM_2/1 -> Transfer Fcn1/1
  PWM_3/1 -> Transfer Fcn2/1
  PWM_4/1 -> Transfer Fcn3/1
  Transfer Fcn4/1 -> Math Function/1
  Transfer Fcn1/1 -> Math Function1/1
  Transfer Fcn2/1 -> Math Function2/1
  Transfer Fcn3/1 -> Math Function3/1
  Gain/1 -> Saturation/1
  Saturation/1 -> M1/1
  Saturation1/1 -> M2/1
  Saturation2/1 -> M3/1
  Saturation3/1 -> M4/1
  Gain1/1 -> Saturation1/1
  Gain2/1 -> Saturation2/1
  Gain3/1 -> Saturation3/1
  Math Function/1 -> Gain/1
  Math Function1/1 -> Gain1/1
  Math Function2/1 -> Gain2/1
  Math Function3/1 -> Gain3/1

== system UAV/Vehicle Interface/Sim_Plant_Model/Battery ==
  PWM_1 : Inport
  PWM_2 : Inport  Port=2
  PWM_3 : Inport  Port=3
  PWM_4 : Inport  Port=4
  " " : Gain  Gain=1/3600
  "  " : Gain  Gain=Drone.Battery.R_internal
  1-D Lookup Table : Lookup_n-D  NumberOfTableDimensions=1  BreakpointsForDimension1=Drone.Battery.DischargeCurve_Cap  Table=Drone.Battery.DischargeCurve_Vol  InternalRulePriority=Speed  RndMeth=Simplest
  Add : Sum  Inputs=++++
  Capacidad : Constant  Value=Drone.Battery.Capacity_Ah
  Divide : Product  Inputs=/*
  I_base : Bias  Bias=Drone.Battery.I_base  SaturateOnIntegerOverflow=off
  I_max : Gain  Gain=Drone.Battery.I_max_motor
  Integrator : Integrator
  Product : Product
  Product1 : Product
  Sum : Sum  Inputs=|+-
  Sum1 : Sum  Inputs=|+-
  Switch : Constant
  Transfer Fcn{1..4} (4 alike) : TransferFcn  Denominator=[0.1 1]
  Battery_Volt : Outport
  Battery_Curr : Outport  Port=2
  wires:
  Transfer Fcn1/1 -> Add/2
  Transfer Fcn3/1 -> Add/4
  Add/1 -> I_max/1
  Transfer Fcn4/1 -> Add/1
  Transfer Fcn2/1 -> Add/3
  PWM_1/1 -> Transfer Fcn4/1
  PWM_2/1 -> Transfer Fcn1/1
  PWM_3/1 -> Transfer Fcn2/1
  PWM_4/1 -> Transfer Fcn3/1
  I_max/1 -> I_base/1
  Integrator/1 -> " "/1
  Capacidad/1 -> Divide/1, Sum/1
  " "/1 -> Sum/2
  Sum/1 -> Divide/2
  Divide/1 -> 1-D Lookup Table/1
  1-D Lookup Table/1 -> Sum1/1
  "  "/1 -> Sum1/2
  I_base/1 -> Product1/2, "  "/1, Integrator/1
  Switch/1 -> Product1/1, Product/2
  Product1/1 -> Battery_Curr/1
  Product/1 -> Battery_Volt/1
  Sum1/1 -> Product/1

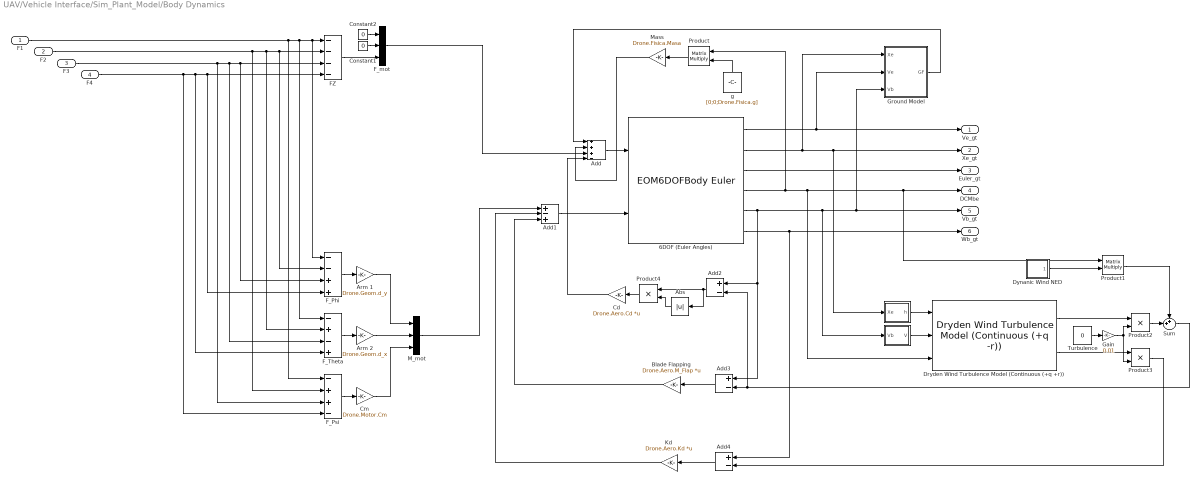
== system UAV/Vehicle Interface/Sim_Plant_Model/Body Dynamics ==
  F1 : Inport
  F2 : Inport  Port=2
  F3 : Inport  Port=3
  F4 : Inport  Port=4
  " " : Subsystem
  "  " : Subsystem
  6DOF (Euler Angles) : EOM6DOFBodyEuler  xme_0=Env.Pos.Init_NED  mass_0=Drone.Fisica.Masa  inertia=Drone.Fisica.InertiaMatrix
  Abs : Abs  SaturateOnIntegerOverflow=off
  Add : Sum  Inputs=+++-
  Add1 : Sum  Inputs=+-+
  Add2 : Sum  Inputs=+-
  Add3 : Sum  Inputs=+-
  Add4 : Sum  Inputs=+-
  Arm 1 : Gain  Gain=Drone.Geom.d_y
  Arm 2 : Gain  Gain=Drone.Geom.d_x
  Blade Flapping : Gain  Gain=Drone.Aero.M_Flap  Multiplication=Matrix(K*u) (u vector)
  Cd : Gain  Gain=Drone.Aero.Cd  Multiplication=Matrix(K*u) (u vector)
  Cm : Gain  Gain=Drone.Motor.Cm
  Constant1 : Constant  Value=0
  Constant2 : Constant  Value=0
  Dryden Wind Turbulence Model (Continuous (+q +r)) : aerolibwind2/Dryden Wind Turbulence Model  (Continuous (+q -r))  units=Metric (MKS)  spec=MIL-F-8785C  model=Continuous Dryden (+q +r)  W20=Env.Viento.Intensidad_Max  Wdeg=0  TurbProb=10^-2 - Light  L_high=533.4  Wingspan=0.318  ts=1/100  Seed=[23341 23342 23343 23344]  T_on=on
      settings: LibrarySourceBlock=|
      | aerolibwind2/Dryden Wind Turbulence Model
      | (Continuous (+q +r))
  Dynanic Wind NED : Subsystem
  FZ : Sum  Inputs=----
  F_Phi : Sum  Inputs=--++
  F_Psi : Sum  Inputs=-++-
  F_Theta : Sum  Inputs=-+-+
  F_mot : Mux  Inputs=3
  Gain : Gain  Gain=0.01
  Ground Model : Subsystem
  Kd : Gain  Gain=Drone.Aero.Kd  Multiplication=Matrix(K*u) (u vector)
  M_mot : Mux  Inputs=3
  Mass : Gain  Gain=Drone.Fisica.Masa
  Product : Product  Multiplication=Matrix(*)
  Product1 : Product  Multiplication=Matrix(*)
  Product2 : Product
  Product3 : Product
  Product4 : Product
  Sum : Sum  Inputs=++|
  Turbulence : Constant  Value=0
  g : Constant  Value=[0;0;Drone.Fisica.g]
  Ve_gt : Outport
  Xe_gt : Outport  Port=2
  Euler_gt : Outport  Port=3
  DCMbe : Outport  Port=4
  Vb_gt : Outport  Port=5
  Wb_gt : Outport  Port=6
  wires:
  F_Phi/1 -> Arm 1/1
  F_Psi/1 -> Cm/1
  F_Theta/1 -> Arm 2/1
  F4/1 -> F_Psi/4, F_Theta/4, F_Phi/4, FZ/4
  F3/1 -> F_Psi/3, F_Theta/3, F_Phi/3, FZ/3
  F2/1 -> F_Psi/2, F_Theta/2, F_Phi/2, FZ/2
  F1/1 -> F_Psi/1, F_Theta/1, F_Phi/1, FZ/1
  Constant1/1 -> F_mot/2
  Constant2/1 -> F_mot/1
  Arm 1/1 -> M_mot/1
  Arm 2/1 -> M_mot/2
  Cm/1 -> M_mot/3
  6DOF (Euler Angles)/6 -> Add4/1, Wb_gt/1
  6DOF (Euler Angles)/5 -> Add2/1, Add3/1, " "/1(Vb), Ground Model/3(Vb), Vb_gt/1
  Add/1 -> 6DOF (Euler Angles)/1
  Add1/1 -> 6DOF (Euler Angles)/2
  M_mot/1 -> Add1/1
  Blade Flapping/1 -> Add1/3
  Kd/1 -> Add1/2
  F_mot/1 -> Add/3
  Cd/1 -> Add/4
  Product/1 -> Mass/1
  Mass/1 -> Add/2
  g/1 -> Product/2
  6DOF (Euler Angles)/4 -> Dryden Wind Turbulence Model (Continuous (+q +r))/3, Product1/1, DCMbe/1, Product/1
  6DOF (Euler Angles)/1 -> Ve_gt/1, Ground Model/2(Ve)
  6DOF (Euler Angles)/3 -> Euler_gt/1
  Ground Model/1(GF) -> Add/1
  6DOF (Euler Angles)/2 -> "  "/1(Xe), Xe_gt/1, Ground Model/1(Xe)
  FZ/1 -> F_mot/3
  " "/1(V) -> Dryden Wind Turbulence Model (Continuous (+q +r))/2
  "  "/1(h) -> Dryden Wind Turbulence Model (Continuous (+q +r))/1
  Dryden Wind Turbulence Model (Continuous (+q +r))/1 -> Product2/1
  Add3/1 -> Blade Flapping/1
  Add4/1 -> Kd/1
  Dryden Wind Turbulence Model (Continuous (+q +r))/2 -> Product3/1
  Product1/1 -> Sum/1
  Product2/1 -> Sum/2
  Sum/1 -> Add2/2, Add3/2
  Dynanic Wind NED/1(Out1) -> Product1/2
  Turbulence/1 -> Gain/1
  Gain/1 -> Product2/2, Product3/2
  Product3/1 -> Add4/2
  Product4/1 -> Cd/1
  Add2/1 -> Abs/1, Product4/1
  Abs/1 -> Product4/2

== system UAV/Vehicle Interface/Sim_Plant_Model/ESC_Quantization_Model ==
  In1 : Inport
  Bias : Bias  Bias=1000  SaturateOnIntegerOverflow=off
  Bias1 : Bias  Bias=-1000  SaturateOnIntegerOverflow=off
  Data Type Conversion : DataTypeConversion  OutDataTypeStr=uint16  SaturateOnIntegerOverflow=off  RndMeth=Floor  LockScale=on
  Data Type Conversion1 : DataTypeConversion  OutDataTypeStr=double  SaturateOnIntegerOverflow=off  RndMeth=Floor  LockScale=on
  Gain : Gain  Gain=1000
  Gain1 : Gain  Gain=1/1000
  Out1 : Outport
  wires:
  Bias/1 -> Data Type Conversion/1
  Data Type Conversion/1 -> Data Type Conversion1/1
  Bias1/1 -> Gain1/1
  Data Type Conversion1/1 -> Bias1/1
  Gain1/1 -> Out1/1
  Gain/1 -> Bias/1
  In1/1 -> Gain/1

== system UAV/Vehicle Interface/Sim_Plant_Model/Flight Recorder ==
  Nav_Data : Inport
  PID_Effort : Inport  Port=2
  Motor_PWM : Inport  Port=3
  To Workspace : ToWorkspace  VariableName=Log_Nav  SaveFormat=Structure With Time  SampleTime=-1
  To Workspace1 : ToWorkspace  VariableName=PID_Effort  SaveFormat=Structure With Time  SampleTime=-1
  To Workspace2 : ToWorkspace  VariableName=Motor_PWM  SaveFormat=Structure With Time  SampleTime=-1
  wires:
  PID_Effort/1 -> To Workspace1/1
  Motor_PWM/1 -> To Workspace2/1
  Nav_Data/1 -> To Workspace/1

== system UAV/Vehicle Interface/Sim_Plant_Model/Sensors ==
  Ve : Inport
  Xe : Inport  Port=2
  Euler : Inport  Port=3
  DCMbe : Inport  Port=4
  Vb : Inport  Port=5
  Wb : Inport  Port=6
  Barometer : Subsystem
  GPS : Subsystem
  IMU : Subsystem
  Magnetometer : Subsystem
  Ve_m : Outport
  Xe_m : Outport  Port=2
  z_m : Outport  Port=3
  Mag_m : Outport  Port=4
  Gyro_m : Outport  Port=5
  Acc_m : Outport  Port=6
  "Euler_gt " : Outport  Port=7
  "Vb_gt " : Outport  Port=8
  Xe_gt : Outport  Port=9
  Ve_gt : Outport  Port=10
  wires:
  Euler/1 -> "Euler_gt "/1
  DCMbe/1 -> IMU/1(DCMbe), Magnetometer/1(DCMbe)
  Vb/1 -> IMU/2(Vb_gt), "Vb_gt "/1
  Wb/1 -> IMU/3(Wb_gt)
  IMU/2(Gyro_m) -> Gyro_m/1
  IMU/1(Acc_m) -> Acc_m/1
  Xe/1 -> Barometer/1(Xe), Xe_gt/1, GPS/2(Xe)
  Ve/1 -> Ve_gt/1, GPS/1(Ve)
  GPS/1(Ve_m) -> Ve_m/1
  GPS/2(Xe_m) -> Xe_m/1
  Barometer/1(z_m) -> z_m/1
  Magnetometer/1(Mag_m) -> Mag_m/1

== system UAV/Vehicle Interface/Sim_Plant_Model/Visualization ==
  Ground Truth : Inport
  Bus Selector : BusSelector  OutputSignals=Xe_gt,Euler_gt
  NED to ENU : Subsystem
  Simulation 3D Scene Configuration : sim3dlib/Simulation 3D Scene Configuration  Priority=0  ProjectFormat=Default Scenes  SceneDesc=US city block  ProjectName=C:\Program Files\MATLAB\R2025b\toolbox\shared\sim3d_projects\automotive_project_windows\UE\WindowsNoEditor\VehicleSimulation.exe  ScenePath=/Game/Maps/USCityBlock  EnableOpenDRIVE=off  vehTagList={'Custom';'Scene Origin'}  vehTag=Scene Origin  AttachedCameraRelativeTranslation=[0 0 0]  FreeCameraDefaultInitialTranslation=[-6, 0, 2]  AttachedCameraRelativeRotation=[0 0 0]  FreeCameraDefaultInitialRotation=[0, -15, 0]  ViewpointName=Custom  FreeCameraInitialTranslation=[0, 0, 0]  ViewpointTranslation=[0, 0, 0]  FreeCameraInitialRotation=[0, 0, 0]  ViewpointRotation=[0, 0, 0]  OpVisEn=off  Ts=1/50  EnableWindow=on  EnableRemoteAccess=off  EnableWeather=off  SunAzimuth=90  SunAltitude=40.0  EnableGeospatialSun=off  Latitude=0  Longitude=0  Date=2023-01-01  Time=10:30:00  GeoTimeZone=-5.0  SunDaylightSaving=off  wind=1  clouds=10  EnableVolumetricClouds=off  CloudCoverage=0  CloudAltitude=6  fog=0  rain=0  RaindropsEffect=off  SnowDensity=0  EnableGeospatial=off  TilesetSource=Earth terrain  UseTrueOrigin=off  OriginHeight=200  OriginLatitude=40.744652  OriginLongitude=-73.988864  MapStyle=Aerial  AdditionalAssetIDs=[]  UseAdvancedSunSky=off  SolarTime=11  TimeZone=-5  Day=21  Month=9  Year=2022  UseDaylightSavingTime=on  DSTStartDay=10  DSTStartMonth=3  DSTEndDay=3  DSTEndMonth=11  DSTSwitchHour=2  sensorTag=MainCamera1  sensorId=1  sensorName=MainCamera1  mountLoc=Origin  offsetFlag=off  tmountOffset=[0, 0, 0]  rmountOffset=[0, 0, 0]  HorizontalResolution=1280  VerticalResolution=720  HorizontalFOV=60  mountPoint=[0 0 0]  mountOrientation=[0 0 0]  aMode=4  ID=1  GeoTrigger=Inactive  ViewNameList={'Custom'}  ViewTranslationList={'[0 0 0]'}  ViewRotationList={'[0 0 0]'}
      settings: LibrarySourceBlock=uavsim3dlib/Simulation 3D Scene Configuration
  Simulation 3D UAV Vehicle1 : uavsim3dlib/Simulation 3D UAV Vehicle  Priority=-1  Mesh=Quadrotor  MeshPath=/MathWorksUAVContent/UAVs/Quadrotor/Quadrotor.Quadrotor  Color=Black  ActorName=SimulinkVehicle1  UseGlobalFrame=off  InitialTranslation=[0 0 0]  InitialRotation=[0 0 0]  InitialTranslationGlobal=[0 0 0]  InitialGeoOrigin=[0 0 0]  InitialRotationGlobal=[0 0 0]  SampleTime=1/50  ActorType=SimulinkVehicle  ID=1  aMode=4  ActorTag=SimulinkVehicle1
  wires:
  NED to ENU/1(T_ENU) -> Simulation 3D UAV Vehicle1/1
  NED to ENU/2(R_ENU) -> Simulation 3D UAV Vehicle1/2
  Ground Truth/1 -> Bus Selector/1
  Bus Selector/1 -> NED to ENU/1(T_NED)  "<Xe_gt>"
  Bus Selector/2 -> NED to ENU/2(R_NED)  "<Euler_gt>"

== system UAV/Flight Controller Software/Flight Controller Software MIL/Flight Supervisor/Batery_Monitor ==
  In1 : Inport
  In2 : Inport  Port=2
  "  " : Gain  Gain=Drone.Battery.R_internal
  1-D Lookup Table : Lookup_n-D  NumberOfTableDimensions=1  BreakpointsForDimension1=Drone.Battery.DischargeCurve_Vol  Table=Drone.Battery.DischargeCurve_Cap * 100  ExtrapMethod=Clip  InternalRulePriority=Speed  RndMeth=Simplest
  Discrete Transfer Fcn : DiscreteTransferFcn  Numerator=[0.01]  Denominator=[1 -0.99]
  Discrete Transfer Fcn1 : DiscreteTransferFcn  Numerator=[0.01]  Denominator=[1 -0.99]
  Sum : Sum  Inputs=|++
  Out1 : Outport
  Out2 : Outport  Port=2
  wires:
  In1/1 -> Discrete Transfer Fcn1/1, Sum/1
  Discrete Transfer Fcn/1 -> 1-D Lookup Table/1
  In2/1 -> "  "/1
  1-D Lookup Table/1 -> Out1/1
  "  "/1 -> Sum/2
  Sum/1 -> Discrete Transfer Fcn/1
  Discrete Transfer Fcn1/1 -> Out2/1

== system UAV/Flight Controller Software/Flight Controller Software MIL/State Estimator/Subsystem ==
  vel_ned : Inport
  DCMbe : Inport  Port=2
  Demux7 : Demux  Outputs=3
  Demux9 : Demux  Outputs=3
  Mux1 : Mux  Inputs=3
  Mux2 : Mux  Inputs=3
  Product : Product  Multiplication=Matrix(*)
  Out1 : Outport
  wires:
  Demux9/2 -> Mux2/2
  Demux9/3 -> Mux1/3
  Demux9/1 -> Mux2/1
  Product/1 -> Demux7/1
  Demux7/2 -> Mux1/2
  Demux7/1 -> Mux1/1
  vel_ned/1 -> Demux9/1
  Mux2/1 -> Product/2
  DCMbe/1 -> Product/1
  Mux1/1 -> Out1/1

== system UAV/Pilot Interface/Real_Receiver_Driver /Command Acquisition/Subsystem ==
  In1 : Inport
  Dead Zone{,1..4} (5 alike) : DeadZone  LowerValue=-0.05  UpperValue=0.05
  Demux : Demux  Outputs=5
  Selector : Selector  InputPortWidth=5  IndexOptions=Index vector (dialog)  Indices=[1 2 3 4 5]  OutputSizes=1
  Zero-Order Hold : ZeroOrderHold  SampleTime=1/100
  Roll : Outport
  Pitch : Outport  Port=2
  Yaw : Outport  Port=3
  Cx : Outport  Port=4
  Cy : Outport  Port=5
  wires:
  Demux/5 -> Dead Zone4/1
  Demux/4 -> Dead Zone3/1
  Demux/2 -> Dead Zone1/1
  Demux/3 -> Dead Zone2/1
  Demux/1 -> Dead Zone/1
  In1/1 -> Zero-Order Hold/1
  Selector/1 -> Demux/1
  Zero-Order Hold/1 -> Selector/1
  Dead Zone/1 -> Roll/1
  Dead Zone1/1 -> Pitch/1
  Dead Zone2/1 -> Cx/1
  Dead Zone3/1 -> Cy/1
  Dead Zone4/1 -> Yaw/1

== system UAV/Pilot Interface/Real_Receiver_Driver /Command Acquisition/Subsystem1 ==
  In1 : Inport
  Demux1 : Demux  Outputs=14
  Selector : Selector  InputPortWidth=17  IndexOptions=Index vector (dialog)  Indices=[1 2 3 4 5 6 7 8 9 10 11 12 13 14]  OutputSizes=1
  Zero-Order Hold1 : ZeroOrderHold  SampleTime=1/100
  Trigger : Outport
  A : Outport  Port=2
  B : Outport  Port=3
  "C " : Outport  Port=4
  "D " : Outport  Port=5
  Lever : Outport  Port=6
  H1U : Outport  Port=7
  H1R : Outport  Port=8
  H1D : Outport  Port=9
  H1L : Outport  Port=10
  H2U : Outport  Port=11
  H2R : Outport  Port=12
  H2D : Outport  Port=13
  H2L : Outport  Port=14
  wires:
  In1/1 -> Zero-Order Hold1/1
  Selector/1 -> Demux1/1
  Demux1/1 -> Trigger/1
  Demux1/2 -> A/1
  Demux1/3 -> B/1
  Demux1/4 -> "C "/1
  Demux1/5 -> "D "/1
  Demux1/6 -> Lever/1
  Demux1/7 -> H1U/1
  Demux1/8 -> H1R/1
  Demux1/9 -> H1D/1
  Demux1/10 -> H1L/1
  Demux1/11 -> H2U/1
  Demux1/12 -> H2R/1
  Demux1/13 -> H2D/1
  Demux1/14 -> H2L/1
  Zero-Order Hold1/1 -> Selector/1

== system UAV/Pilot Interface/Real_Receiver_Driver /Command Acquisition/Subsystem2 ==
  In1 : Inport
  Compare To Constant : simulink/Logic and Bit Operations/Compare To Constant  relop===  const=0  OutDataTypeStr=boolean
  Compare To Constant1 : simulink/Logic and Bit Operations/Compare To Constant  relop===  const=90  OutDataTypeStr=boolean
  Compare To Constant2 : simulink/Logic and Bit Operations/Compare To Constant  relop===  const=180  OutDataTypeStr=boolean
  Compare To Constant3 : simulink/Logic and Bit Operations/Compare To Constant  relop===  const=270  OutDataTypeStr=boolean
  Selector : Selector  InputPortWidth=1  IndexOptions=Index vector (dialog)  Indices=[1]  OutputSizes=1
  Zero-Order Hold2 : ZeroOrderHold  SampleTime=1/100
  POV_U : Outport
  POV_R : Outport  Port=2
  POV_D : Outport  Port=3
  POV_L : Outport  Port=4
  wires:
  In1/1 -> Zero-Order Hold2/1
  Zero-Order Hold2/1 -> Selector/1
  Compare To Constant/1 -> POV_U/1
  Compare To Constant1/1 -> POV_R/1
  Compare To Constant2/1 -> POV_D/1
  Compare To Constant3/1 -> POV_L/1
  Selector/1 -> Compare To Constant3/1, Compare To Constant2/1, Compare To Constant1/1, Compare To Constant/1

== system UAV/Pilot Interface/Real_Receiver_Driver /Command Acquisition/Subsystem3 ==
  In1 : Inport
  Dead Zone{,1..7} (8 alike) : DeadZone  LowerValue=-0.05  UpperValue=0.05
  Demux : Demux  Outputs=8
  Selector : Selector  InputPortWidth=8  IndexOptions=Index vector (dialog)  Indices=[1 2 3 4 5 6 7 8]  OutputSizes=1
  Zero-Order Hold : ZeroOrderHold  SampleTime=1/100
  Left TL : Outport
  Right TL : Outport  Port=2
  F : Outport  Port=3
  Cx : Outport  Port=4
  Cy : Outport  Port=5
  G : Outport  Port=6
  RTY 3 : Outport  Port=7
  RTY 4 : Outport  Port=8
  wires:
  Demux/5 -> Dead Zone4/1
  Demux/4 -> Dead Zone3/1
  Demux/2 -> Dead Zone1/1
  Demux/3 -> Dead Zone2/1
  Demux/1 -> Dead Zone/1
  In1/1 -> Zero-Order Hold/1
  Selector/1 -> Demux/1
  Zero-Order Hold/1 -> Selector/1
  Demux/6 -> Dead Zone5/1
  Demux/7 -> Dead Zone6/1
  Demux/8 -> Dead Zone7/1
  Dead Zone1/1 -> Right TL/1
  Dead Zone2/1 -> F/1
  Dead Zone3/1 -> Cx/1
  Dead Zone4/1 -> Cy/1
  Dead Zone5/1 -> G/1
  Dead Zone6/1 -> RTY 3/1
  Dead Zone7/1 -> RTY 4/1
  Dead Zone/1 -> Left TL/1

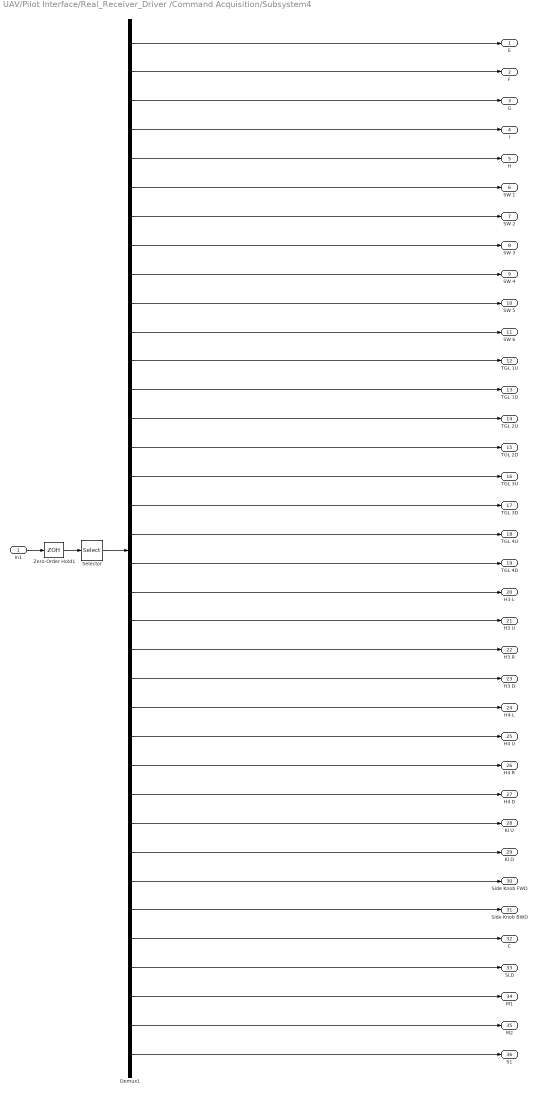
== system UAV/Pilot Interface/Real_Receiver_Driver /Command Acquisition/Subsystem4 ==
  In1 : Inport
  Demux1 : Demux  Outputs=36
  Selector : Selector  InputPortWidth=36  IndexOptions=Index vector (dialog)  Indices=[1 2 3 4 5 6 7 8 9 10 11 12 13 14 15 16 17 18 19 20 21 22 23 24 25 26 27 28 29 30 31 32 33 34 35 36]  OutputSizes=1
  Zero-Order Hold1 : ZeroOrderHold  SampleTime=1/100
  E : Outport
  F : Outport  Port=2
  G : Outport  Port=3
  I : Outport  Port=4
  H : Outport  Port=5
  SW 1 : Outport  Port=6
  SW 2 : Outport  Port=7
  SW 3 : Outport  Port=8
  SW 4 : Outport  Port=9
  SW 5 : Outport  Port=10
  SW 6 : Outport  Port=11
  TGL 1U : Outport  Port=12
  TGL 1D : Outport  Port=13
  TGL 2U : Outport  Port=14
  TGL 2D : Outport  Port=15
  TGL 3U : Outport  Port=16
  TGL 3D : Outport  Port=17
  TGL 4U : Outport  Port=18
  TGL 4D : Outport  Port=19
  H3 L : Outport  Port=20
  H3 U : Outport  Port=21
  H3 R : Outport  Port=22
  H3 D : Outport  Port=23
  H4 L : Outport  Port=24
  H4 U : Outport  Port=25
  H4 R : Outport  Port=26
  H4 D : Outport  Port=27
  KI U : Outport  Port=28
  KI D : Outport  Port=29
  Side Knob FWD : Outport  Port=30
  Side Knob BWD : Outport  Port=31
  C : Outport  Port=32
  SLD : Outport  Port=33
  M1 : Outport  Port=34
  M2 : Outport  Port=35
  S1 : Outport  Port=36
  wires:
  Selector/1 -> Demux1/1
  Zero-Order Hold1/1 -> Selector/1
  In1/1 -> Zero-Order Hold1/1
  Demux1/1 -> E/1
  Demux1/2 -> F/1
  Demux1/3 -> G/1
  Demux1/5 -> H/1
  Demux1/6 -> SW 1/1
  Demux1/7 -> SW 2/1
  Demux1/8 -> SW 3/1
  Demux1/9 -> SW 4/1
  Demux1/13 -> TGL 1D/1
  Demux1/14 -> TGL 2U/1
  Demux1/15 -> TGL 2D/1
  Demux1/16 -> TGL 3U/1
  Demux1/17 -> TGL 3D/1
  Demux1/18 -> TGL 4U/1
  Demux1/19 -> TGL 4D/1
  Demux1/20 -> H3 L/1
  Demux1/21 -> H3 U/1
  Demux1/22 -> H3 R/1
  Demux1/23 -> H3 D/1
  Demux1/24 -> H4 L/1
  Demux1/25 -> H4 U/1
  Demux1/26 -> H4 R/1
  Demux1/27 -> H4 D/1
  Demux1/28 -> KI U/1
  Demux1/29 -> KI D/1
  Demux1/30 -> Side Knob FWD/1
  Demux1/31 -> Side Knob BWD/1
  Demux1/32 -> C/1
  Demux1/33 -> SLD/1
  Demux1/34 -> M1/1
  Demux1/35 -> M2/1
  Demux1/36 -> S1/1
  Demux1/4 -> I/1
  Demux1/10 -> SW 5/1
  Demux1/11 -> SW 6/1
  Demux1/12 -> TGL 1U/1

== system UAV/Pilot Interface/Real_Receiver_Driver /Flight Data Display/Subsystem ==
  seg : Inport
  Compose String : ComposeString  Format="\"%02d:%02d\""
  Constant : Constant  Value=60
  Data Type Conversion : DataTypeConversion  SaturateOnIntegerOverflow=off  RndMeth=Floor
  Data Type Conversion1 : DataTypeConversion  SaturateOnIntegerOverflow=off  RndMeth=Floor
  Floor : Rounding
  Floor1 : Rounding
  Gain : Gain  Gain=1/60
  Math Function : Math  Operator=mod
  MM:SS : Outport
  wires:
  Constant/1 -> Math Function/2
  Gain/1 -> Floor/1
  Floor1/1 -> Data Type Conversion1/1
  Data Type Conversion/1 -> Compose String/1
  Data Type Conversion1/1 -> Compose String/2
  Math Function/1 -> Floor1/1
  Floor/1 -> Data Type Conversion/1
  seg/1 -> Gain/1, Math Function/1
  Compose String/1 -> MM:SS/1
